simulink model "Solar_Seguidor_V2"  (R2021b)
settings: Solver=ode1  StartTime=0.0  StopTime=10  FixedStep=25e-6  RelTol=1e-3
PostLoadFcn:
  | %clc; clear all; close all;
  | %%%%%%%%%%%%%%%%%%%%%%%%%%%%%%%%%%%%%%%%%%%%%%%%
  | %%%%%%%%% Solar seguidor de rede %%%%%%%%%%
  | %%%%%%%%%%%%%%%%%%%%%%%%%%%%%%%%%%%%%%%%%%%%%%%%
  | %%%% Nominal Parameters %%%%
  | Pnom = 16e3;                                         % Potencia Nominal
  | Vnom_rms = 210;                                    % V linha rms
  | Vnom_peak = sqrt(2/3)*Vnom_rms;                     % V fase pico
  | FP_min = 1;                                       % Para suporte de reativo
  | Snom = Pnom/FP_min;                                 % Potencia aparente
  | Irms = Pnom/(sqrt(3)*Vnom_rms);                     % Ig rms
  | Inom_peak = Irms*sqrt(2);                           % Ig pico
  | Zbase = Vnom_peak/Inom_peak;                        % Impedancia Base
  | f = 60;                                             % Freq nominal
  | wnom = 2*pi*60;                                     % Freq Ang. nominal
  | m = 0.805;                                            % Indice mod nominal
  | Vdc = 2*(Vnom_peak/m);                              % Vcc
  | Vdc_2 = Vdc/2;                                      % Metade Vcc
  | Kconv = Zbase;                                      % Ganho conversor
  | %%%% Transformer %%%%
  | S_trafo = 250e3;                                      % transformer apparent power
  | Vrms_high = 400;                                   % transformer secondary voltage - Wye connection
  | Vrms_low = 210;                                   % transformer primary voltage - Delta connection
  | N = Vrms_high/Vrms_low;                             % transformation relationship
  | X_pu_trafo = 0.03;                                 % transformer p.u. reactance
  | Zb_trafo_high = ((Vrms_high)^2)/S_trafo;            % secondary base impedance
  | Zb_trafo = ((Vnom_rms)^2)/S_trafo;                  % primary base impedance
  | L_trafo = (X_pu_trafo*Zb_trafo)/wnom;               % primary inductance
  | %%%% LCL Filter Project %%%%
  | fsw = 105*60;%105*60;                                         % switching frequency
  | ripple = 0.05;                                       % current ripple
  | L1 = Vdc/(6*ripple*Inom_peak*fsw);                  % inductor L1
  |  RL1 = 0.005;                                        % L1 resistance
  |  Cbase = 1/(wnom*Kconv);                             % base capacitance
  |  Cf = 0.05*Cbase;                                    % filter capacitor
  | % Calculo do filtro
  | Sbase = 16e3;
  | %Sbase = 200e3*1.12;
  | V_LL = 210;
  | V_LG = 210/sqrt(3);
  | Vbase = V_LG*sqrt(2);
  | Ibase = (Sbase*sqrt(2))/(V_LG*3)*sqrt(3/2);
  | Zbase = (V_LL^2)/Sbase;
  | Rbase = Zbase;
  | Xbase = Zbase;
  | Lbase = Xbase/(2*pi*60);
  | Cbase = 1/(Xbase*2*pi*60);
  | w = 2*pi*60;
  | Q = 70;
  | Lf = 0.15*Lbase;
  | Cf = 0.05*Cbase;
  | fc = 1/(2*pi*sqrt(Lf*Cf));
  | R = (w*Lf)/Q;
  | Lf = L1;
  | R = RL1;
  | ka=0.2;                                             % attenuation factor
  | L2 = (sqrt(1/(ka^2))+1)/(Cf*((2*pi*fsw)^2));        % inductor L2
  | RL2 = 0.005;                                        % L2 resistance
  | w_res = sqrt((L1+L2+L_trafo)/(L1*L2*Cf));           % resonant angular frequency
  | f_res = w_res/(2*pi);                               % resonant frequency
  | ... (+31 lines)
InitFcn:
  | %clc; clear all; close all;
  | %%%%%%%%%%%%%%%%%%%%%%%%%%%%%%%%%%%%%%%%%%%%%%%%
  | %%%%%%%%% Solar seguidor de rede %%%%%%%%%%
  | %%%%%%%%%%%%%%%%%%%%%%%%%%%%%%%%%%%%%%%%%%%%%%%%
  | %%%% Nominal Parameters %%%%
  | Pnom = 16e3;                                         % Potencia Nominal
  | Vnom_rms = 210;                                    % V linha rms
  | Vnom_peak = sqrt(2/3)*Vnom_rms;                     % V fase pico
  | FP_min = 1;                                       % Para suporte de reativo
  | Snom = Pnom/FP_min;                                 % Potencia aparente
  | Irms = Pnom/(sqrt(3)*Vnom_rms);                     % Ig rms
  | Inom_peak = Irms*sqrt(2);                           % Ig pico
  | Zbase = Vnom_peak/Inom_peak;                        % Impedancia Base
  | f = 60;                                             % Freq nominal
  | wnom = 2*pi*60;                                     % Freq Ang. nominal
  | m = 0.805;                                            % Indice mod nominal
  | Vdc = 2*(Vnom_peak/m);                              % Vcc
  | Vdc_2 = Vdc/2;                                      % Metade Vcc
  | Kconv = Zbase;                                      % Ganho conversor
  | %%%% Transformer %%%%
  | S_trafo = 250e3;                                      % transformer apparent power
  | Vrms_high = 400;                                   % transformer secondary voltage - Wye connection
  | Vrms_low = 210;                                   % transformer primary voltage - Delta connection
  | N = Vrms_high/Vrms_low;                             % transformation relationship
  | X_pu_trafo = 0.03;                                 % transformer p.u. reactance
  | Zb_trafo_high = ((Vrms_high)^2)/S_trafo;            % secondary base impedance
  | Zb_trafo = ((Vnom_rms)^2)/S_trafo;                  % primary base impedance
  | L_trafo = (X_pu_trafo*Zb_trafo)/wnom;               % primary inductance
  | %%%% LCL Filter Project %%%%
  | fsw = 105*60;%105*60;                                         % switching frequency
  | ripple = 0.05;                                       % current ripple
  | L1 = Vdc/(6*ripple*Inom_peak*fsw);                  % inductor L1
  |  RL1 = 0.005;                                        % L1 resistance
  |  Cbase = 1/(wnom*Kconv);                             % base capacitance
  |  Cf = 0.05*Cbase;                                    % filter capacitor
  | % Calculo do filtro
  | Sbase = 16e3;
  | %Sbase = 200e3*1.12;
  | V_LL = 210;
  | V_LG = 210/sqrt(3);
  | Vbase = V_LG*sqrt(2);
  | Ibase = (Sbase*sqrt(2))/(V_LG*3)*sqrt(3/2);
  | Zbase = (V_LL^2)/Sbase;
  | Rbase = Zbase;
  | Xbase = Zbase;
  | Lbase = Xbase/(2*pi*60);
  | Cbase = 1/(Xbase*2*pi*60);
  | w = 2*pi*60;
  | Q = 70;
  | Lf = 0.15*Lbase;
  | Cf = 0.05*Cbase;
  | fc = 1/(2*pi*sqrt(Lf*Cf));
  | R = (w*Lf)/Q;
  | Lf = L1;
  | R = RL1;
  | ka=0.2;                                             % attenuation factor
  | L2 = (sqrt(1/(ka^2))+1)/(Cf*((2*pi*fsw)^2));        % inductor L2
  | RL2 = 0.005;                                        % L2 resistance
  | w_res = sqrt((L1+L2+L_trafo)/(L1*L2*Cf));           % resonant angular frequency
  | f_res = w_res/(2*pi);                               % resonant frequency
  | ... (+31 lines)
undefined symbols (not defined in the file): D1, Delta, DERS_models, DiscIntNeverNeededParam, eHS, I, Ia_PV, Ib_PV, Ic_PV, Left, parameter_set_id, ph, PV_system, type, V, Va_grid, Vb_grid, Vc_grid
libraries: powerlib_meascontrol x17, rtlab x14, spsThreePhaseSeriesRLCBranchLib x9, spsCurrentMeasurementLib x9, artemis x7, spsThreePhaseVIMeasurementLib x6, slpidlib x6, rteventslib x6, spsabctodq0Lib x4, spsThreePhaseTransformerTwoWindingsLib x3, simulink x3, spsPVArrayLib x3
(part 4 of 4)

== system Solar_Seguidor_V2/SM_mestre1/PV_system2/VSC_Control/Voltage DC Controller ==
  note: Voltage Controller
  Vdc_mes : Inport  PortDimensions=1
  Vdc_ref : Inport  Port=2  PortDimensions=1
  hab : Inport  Port=3
  Id_refm : Scope
  Math Function1 : Math  Operator=square  SaturateOnIntegerOverflow=on
  Math Function2 : Math  Commented=on  Operator=square  SaturateOnIntegerOverflow=on
  Math Function3 : Math  Operator=square  SaturateOnIntegerOverflow=on
  Mux : Mux  Inputs=2
  PI : slpidlib/PID Controller  Commented=on  Controller=PI  Form=Parallel  TimeDomain=Continuous-time  UseExternalTs=off  SampleTime=Ts  IntegratorMethod=Trapezoidal  FilterMethod=Forward Euler  ControllerParametersSource=internal  P=Kp_dc  I=ki_dc_pu  D=0  UseFilter=on  N=100  TunerSelectOption=Transfer Function Based (PID Tuner App)  InitialConditionSource=internal  InitialConditionForIntegrator=0  InitialConditionForFilter=0  DifferentiatorICPrevScaledInput=0  ExternalReset=rising  TrackingMode=off  Kt=1  LimitOutput=on  SatLimitsSource=internal  UpperSaturationLimit=1.4  LowerSaturationLimit=-2  LinearizeAsGain=off  AntiWindupMode=clamping  Kb=1  POutMin=[]  POutMax=[]  IOutMin=[]  IOutMax=[]  DOutMin=[]  DOutMax=[]  NOutMin=[]  NOutMax=[]  SumOutMin=[]  SumOutMax=[]  SaturationOutMin=[]  SaturationOutMax=[]  PParamMin=[]  PParamMax=[]  IParamMin=[]  IParamMax=[]  DParamMin=[]  DParamMax=[]  NParamMin=[]  NParamMax=[]  KbParamMin=[]  KbParamMax=[]  KtParamMin=[]  KtParamMax=[]  KbOutMin=[]  KbOutMax=[]  KtOutMin=[]  KtOutMax=[]  IntegratorOutMin=[]  IntegratorOutMax=[]  FilterOutMin=[]  FilterOutMax=[]  SumI1OutMin=[]  SumI1OutMax=[]  SumI2OutMin=[]  SumI2OutMax=[]  SumI3OutMin=[]  SumI3OutMax=[]  SumI4OutMin=[]  SumI4OutMax=[]  SumDOutMin=[]  SumDOutMax=[]  DifferentiatorOutMin=[]  DifferentiatorOutMax=[]  FilterDiffOutCoefMin=[]  FilterDiffOutCoefMax=[]  ReciprocalOutMin=[]  ReciprocalOutMax=[]  SumDenOutMin=[]  SumDenOutMax=[]  SumNumOutMin=[]  SumNumOutMax=[]  DivideOutMin=[]  DivideOutMax=[]  UdiffTsProdOutMin=[]  UdiffTsProdOutMax=[]  NTsProdOutMin=[]  NTsProdOutMax=[]  UintegralTsProdOutMin=[]  UintegralTsProdOutMax=[]  UngainTsProdOutMin=[]  UngainTsProdOutMax=[]  FilterDenConstantOutDataTypeStr=Inherit: Inherit via back propagation  FilterDenConstantOutMin=[]  FilterDenConstantOutMax=[]  PCopyOutDataTypeStr=Inherit: Inherit via back propagation  PCopyOutMin=[]  PCopyOutMax=[]  NCopyOutDataTypeStr=Inherit: Inherit via back propagation  NCopyOutMin=[]  NCopyOutMax=[]  IntegratorContinuousStateAttributes=''  IntegratorStateMustResolveToSignalObject=off  IntegratorRTWStateStorageClass=Auto  FilterContinuousStateAttributes=''  FilterStateMustResolveToSignalObject=off  FilterRTWStateStorageClass=Auto  ParallelPVariant=InternalParameters  IdealPVariant=Disabled  IVariant=InternalParameters  DVariant=Disabled  IntegratorVariant=Continuous  SatVariant=Enabled  AWVariant=ContClampingParallel  PCopyVariant=Disabled  TRVariant=Disabled  FdbkBlocksVariant=Forward  IdealPFdbkVariant=Disabled  SatFdbkVariant=Disabled  DerivativeFilterVariant=Disabled  NVariant=Disabled  NCopyVariant=Disabled_SignalSpec  FilterICVariant=Disabled  IntegratorICVariant=InternalICs  ExternalResetVariant=ExternalReset  TRSumVariant=Passthrough  SumFdbkVariant=Disabled  SumVariant=Sum_PI  TsampFilterVariant=InternalTs  TsampNgainVariant=Passthrough  TsampIntegralVariant=Passthrough  ExternalSaturationOutDataTypeStr=Inherit: Same as second input
  PI_Vdc2 : Subsystem
  Product : Product
  Rtot_pu1 : Gain  Gain=1/430  SaturateOnIntegerOverflow=on  OutDataTypeStr=Inherit: Same as input  ParamDataTypeStr=Inherit: Same as input
  Rtot_pu2 : Gain  Gain=1/430  SaturateOnIntegerOverflow=on  OutDataTypeStr=Inherit: Same as input  ParamDataTypeStr=Inherit: Same as input
  Rtot_pu3 : Gain  Gain=-1  SaturateOnIntegerOverflow=on  OutDataTypeStr=Inherit: Same as input  ParamDataTypeStr=Inherit: Same as input
  Saturation : Saturate  UpperLimit=1.2  LowerLimit=0
  Sum : Sum  Inputs=|-+
  Transfer Fcn2 : TransferFcn  Denominator=[2.53e-4 1]
  Voltage_DC : Scope
  Id_ref : Outport  SampleTime=Ts  InitialOutput=0  VectorParamsAs1DForOutWhenUnconnected=off
  wires:
  Saturation/1 -> Id_ref/1
  Vdc_mes/1 -> Transfer Fcn2/1
  Math Function3/1 -> Sum/2
  Math Function1/1 -> Sum/1
  Rtot_pu2/1 -> Math Function3/1, Mux/2
  Rtot_pu1/1 -> Math Function1/1, Mux/1
  Mux/1 -> Voltage_DC/1
  hab/1 -> Product/2, PI_Vdc2/2(hab)
  Sum/1 -> Rtot_pu3/1
  Vdc_ref/1 -> Rtot_pu2/1
  Rtot_pu3/1 -> PI_Vdc2/1(e_Vdc)
  Transfer Fcn2/1 -> Rtot_pu1/1
  PI_Vdc2/1(u) -> Product/1
  Product/1 -> Id_refm/1, Saturation/1

== system Solar_Seguidor_V2/SM_mestre1/PV_system/VSC_Control/Maximum Power Point/MPPT Parameters ==
  Lower limit for Vdc_ref (Dmax) : Constant  Value=375
  Mux9 : Mux
  Upper limit for Vdc_ref (Dmax : Constant  Value=430
  Vdc_ref (DeltaD) : Constant  Value=3e-4*0.5
  Vdc_ref output (Dinit) : Constant  Value=425
  Param : Outport  VectorParamsAs1DForOutWhenUnconnected=off
  wires:
  Upper limit for Vdc_ref (Dmax/1 -> Mux9/2
  Lower limit for Vdc_ref (Dmax)/1 -> Mux9/3
  Vdc_ref output (Dinit)/1 -> Mux9/1
  Mux9/1 -> Param/1
  Vdc_ref (DeltaD)/1 -> Mux9/4

== system Solar_Seguidor_V2/SM_mestre1/PV_system/VSC_Control/PLL & dq/Subsystem ==
  wt : Inport
  Vabc : Inport  Port=2
  Iabc : Inport  Port=3
  Demux : Demux  Outputs=3
  Demux1 : Demux  Outputs=3
  Gain : Gain  Gain=3/2
  Gain1 : Gain  Gain=1/1e3
  Product : Product
  Product1 : Product
  Sum : Sum
  Transfer Fcn : TransferFcn  Denominator=[3/4 1]
  abc to dq1 : powerlib_meascontrol/Transformations/abc to dq0  Alignment=90 degrees behind phase A axis
  abc to dq2 : powerlib_meascontrol/Transformations/abc to dq0  Alignment=90 degrees behind phase A axis
  P_PV : Outport
  wires:
  [Id] -> Product/2
  Product/1 -> Sum/1
  Gain1/1 -> Transfer Fcn/1
  [Vd] -> Product/1
  Gain/1 -> Gain1/1
  [Iq] -> Product1/2
  Sum/1 -> Gain/1
  Product1/1 -> Sum/2
  Transfer Fcn/1 -> P_PV/1
  [Vq] -> Product1/1
  Vabc/1 -> abc to dq1/1
  wt/1 -> abc to dq2/2, abc to dq1/2
  Iabc/1 -> abc to dq2/1
  abc to dq1/1 -> Demux/1
  Demux/1 -> [Vd]
  Demux/2 -> [Vq]
  Demux1/2 -> [Iq]
  Demux1/1 -> [Id]
  abc to dq2/1 -> Demux1/1

== system Solar_Seguidor_V2/SM_mestre1/PV_system1/VSC_Control/Maximum Power Point/MPPT Parameters ==
  Lower limit for Vdc_ref (Dmax) : Constant  Value=375
  Mux9 : Mux
  Upper limit for Vdc_ref (Dmax : Constant  Value=430
  Vdc_ref (DeltaD) : Constant  Value=3e-4*0.5
  Vdc_ref output (Dinit) : Constant  Value=425
  Param : Outport  VectorParamsAs1DForOutWhenUnconnected=off
  wires:
  Vdc_ref (DeltaD)/1 -> Mux9/4
  Mux9/1 -> Param/1
  Vdc_ref output (Dinit)/1 -> Mux9/1
  Lower limit for Vdc_ref (Dmax)/1 -> Mux9/3
  Upper limit for Vdc_ref (Dmax/1 -> Mux9/2

== system Solar_Seguidor_V2/SM_mestre1/PV_system1/VSC_Control/PLL & dq/Subsystem ==
  wt : Inport
  Vabc : Inport  Port=2
  Iabc : Inport  Port=3
  Demux : Demux  Outputs=3
  Demux1 : Demux  Outputs=3
  Gain : Gain  Gain=3/2
  Gain1 : Gain  Gain=1/1e3
  Product : Product
  Product1 : Product
  Sum : Sum
  Transfer Fcn : TransferFcn  Denominator=[3/4 1]
  abc to dq1 : powerlib_meascontrol/Transformations/abc to dq0  Alignment=90 degrees behind phase A axis
  abc to dq2 : powerlib_meascontrol/Transformations/abc to dq0  Alignment=90 degrees behind phase A axis
  P_PV : Outport
  wires:
  abc to dq2/1 -> Demux1/1
  Demux1/1 -> [Id]
  Demux1/2 -> [Iq]
  Demux/2 -> [Vq]
  Demux/1 -> [Vd]
  abc to dq1/1 -> Demux/1
  Iabc/1 -> abc to dq2/1
  wt/1 -> abc to dq1/2, abc to dq2/2
  Vabc/1 -> abc to dq1/1
  [Vq] -> Product1/1
  Transfer Fcn/1 -> P_PV/1
  Product1/1 -> Sum/2
  Sum/1 -> Gain/1
  [Iq] -> Product1/2
  Gain/1 -> Gain1/1
  [Vd] -> Product/1
  Gain1/1 -> Transfer Fcn/1
  Product/1 -> Sum/1
  [Id] -> Product/2

== system Solar_Seguidor_V2/SM_mestre1/PV_system2/VSC_Control/Current Controller/PI_Idq1 ==
  e_Idq : Inport
  hab : Inport  Port=2
  Discrete-Time Integrator : DiscreteIntegrator  SampleTime=-1  ICPrevOutput=DiscIntNeverNeededParam  ICPrevScaledInput=DiscIntNeverNeededParam
  Gain1 : Gain  Gain=kp_current_pu
  Gain2 : Gain  Gain=ki_current_pu
  Product : Product
  Sum1 : Sum
  u : Outport
  wires:
  hab/1 -> Product/2
  e_Idq/1 -> Product/1
  Discrete-Time Integrator/1 -> Sum1/2
  Sum1/1 -> u/1
  Gain1/1 -> Sum1/1
  Product/1 -> Gain2/1, Gain1/1
  Gain2/1 -> Discrete-Time Integrator/1

== system Solar_Seguidor_V2/SM_mestre1/PV_system2/VSC_Control/Maximum Power Point/MPPT Parameters ==
  Lower limit for Vdc_ref (Dmax) : Constant  Value=375
  Mux9 : Mux
  Upper limit for Vdc_ref (Dmax : Constant  Value=430
  Vdc_ref (DeltaD) : Constant  Value=3e-4*0.5
  Vdc_ref output (Dinit) : Constant  Value=425
  Param : Outport  VectorParamsAs1DForOutWhenUnconnected=off
  wires:
  Vdc_ref (DeltaD)/1 -> Mux9/4
  Mux9/1 -> Param/1
  Vdc_ref output (Dinit)/1 -> Mux9/1
  Lower limit for Vdc_ref (Dmax)/1 -> Mux9/3
  Upper limit for Vdc_ref (Dmax/1 -> Mux9/2

== system Solar_Seguidor_V2/SM_mestre1/PV_system2/VSC_Control/PLL & dq/Subsystem ==
  wt : Inport
  Vabc : Inport  Port=2
  Iabc : Inport  Port=3
  Demux : Demux  Outputs=3
  Demux1 : Demux  Outputs=3
  Gain : Gain  Gain=3/2
  Gain1 : Gain  Gain=1/1e3
  Product : Product
  Product1 : Product
  Sum : Sum
  Transfer Fcn : TransferFcn  Denominator=[3/4 1]
  abc to dq1 : spsabctodq0Lib/abc to dq0  Alignment=90 degrees behind phase A axis
  abc to dq2 : spsabctodq0Lib/abc to dq0  Alignment=90 degrees behind phase A axis
  P_PV : Outport
  wires:
  abc to dq2/1 -> Demux1/1
  Demux1/1 -> [Id]
  Demux1/2 -> [Iq]
  Demux/2 -> [Vq]
  Demux/1 -> [Vd]
  abc to dq1/1 -> Demux/1
  Iabc/1 -> abc to dq2/1
  wt/1 -> abc to dq1/2, abc to dq2/2
  Vabc/1 -> abc to dq1/1
  [Vq] -> Product1/1
  Transfer Fcn/1 -> P_PV/1
  Product1/1 -> Sum/2
  Sum/1 -> Gain/1
  [Iq] -> Product1/2
  Gain/1 -> Gain1/1
  [Vd] -> Product/1
  Gain1/1 -> Transfer Fcn/1
  Product/1 -> Sum/1
  [Id] -> Product/2

== system Solar_Seguidor_V2/SM_mestre1/PV_system2/VSC_Control/Voltage DC Controller/PI_Vdc2 ==
  e_Vdc : Inport
  hab : Inport  Port=2
  Discrete-Time Integrator : DiscreteIntegrator  SampleTime=-1  ICPrevOutput=DiscIntNeverNeededParam  ICPrevScaledInput=DiscIntNeverNeededParam
  Gain1 : Gain  Gain=Kp_dc
  Gain2 : Gain  Gain=ki_dc_pu
  Product : Product
  Sum1 : Sum
  u : Outport
  wires:
  Gain2/1 -> Discrete-Time Integrator/1
  Product/1 -> Gain1/1, Gain2/1
  Gain1/1 -> Sum1/1
  Sum1/1 -> u/1
  Discrete-Time Integrator/1 -> Sum1/2
  e_Vdc/1 -> Product/1
  hab/1 -> Product/2

== matlab function Solar_Seguidor_V2/SM_mestre1/PV_system/VSC_Control/Maximum Power Point/MPPT Controller using Perturbe & Observe technique 2 ==
  settings: updateMethod=DISCRETE  sampleTime=Ts*2
  data: Param input; Enabled input; V input; I input; D output
function D  = PandO(Param, Enabled, V, I)

% MPPT controller based on the Perturb & Observe algorithm.

% D output = Reference for DC link voltage (Vdc_ref) 
%
% Enabled input = 1 to enable the MPPT controller
% V input = PV array terminal voltage (V)
% I input = PV array current (A)
%
% Param input:
Dinit = Param(1);  %Initial value for Vdc_ref
Dmax = Param(2);   %Maximum value for Vdc_ref
Dmin = Param(3);   %Minimum value for Vdc_ref
deltaD = Param(4); %Increment value used to increase/decrease Vdc_ref
%  

persistent Vold Pold Dold;

dataType = 'double';

if isempty(Vold)
    Vold=0;
    Pold=0;
    Dold=Dinit;
end
P= V*I;
dV= V - Vold;
dP= P - Pold;

if dP ~= 0 & Enabled ~=0
    if dP < 0
        if dV < 0
            D = Dold + deltaD;
        else
            D = Dold - deltaD;
        end
    else
        if dV < 0
            D = Dold - deltaD;
        else
            D = Dold + deltaD;
        end    
    end
else D=Dold;
end

if D >= Dmax | D<= Dmin
    D=Dold;
end

Dold=D;
Vold=V;
Pold=P;

== matlab function Solar_Seguidor_V2/SM_mestre1/PV_system1/VSC_Control/Maximum Power Point/MPPT Controller using Perturbe & Observe technique 2 ==
  settings: updateMethod=DISCRETE  sampleTime=Ts*2
  data: Param input; Enabled input; V input; I input; D output
function D  = PandO(Param, Enabled, V, I)

% MPPT controller based on the Perturb & Observe algorithm.

% D output = Reference for DC link voltage (Vdc_ref) 
%
% Enabled input = 1 to enable the MPPT controller
% V input = PV array terminal voltage (V)
% I input = PV array current (A)
%
% Param input:
Dinit = Param(1);  %Initial value for Vdc_ref
Dmax = Param(2);   %Maximum value for Vdc_ref
Dmin = Param(3);   %Minimum value for Vdc_ref
deltaD = Param(4); %Increment value used to increase/decrease Vdc_ref
%  

persistent Vold Pold Dold;

dataType = 'double';

if isempty(Vold)
    Vold=0;
    Pold=0;
    Dold=Dinit;
end
P= V*I;
dV= V - Vold;
dP= P - Pold;

if dP ~= 0 & Enabled ~=0
    if dP < 0
        if dV < 0
            D = Dold + deltaD;
        else
            D = Dold - deltaD;
        end
    else
        if dV < 0
            D = Dold - deltaD;
        else
            D = Dold + deltaD;
        end    
    end
else D=Dold;
end

if D >= Dmax | D<= Dmin
    D=Dold;
end

Dold=D;
Vold=V;
Pold=P;

== matlab function Solar_Seguidor_V2/SM_mestre1/PV_system2/VSC_Control/Maximum Power Point/MPPT Controller using Perturbe & Observe technique 2 ==
  settings: updateMethod=DISCRETE  sampleTime=Ts*2
  data: Param input; Enabled input; V input; I input; D output
function D  = PandO(Param, Enabled, V, I)

% MPPT controller based on the Perturb & Observe algorithm.

% D output = Reference for DC link voltage (Vdc_ref) 
%
% Enabled input = 1 to enable the MPPT controller
% V input = PV array terminal voltage (V)
% I input = PV array current (A)
%
% Param input:
Dinit = Param(1);  %Initial value for Vdc_ref
Dmax = Param(2);   %Maximum value for Vdc_ref
Dmin = Param(3);   %Minimum value for Vdc_ref
deltaD = Param(4); %Increment value used to increase/decrease Vdc_ref
%  

persistent Vold Pold Dold;

dataType = 'double';

if isempty(Vold)
    Vold=0;
    Pold=0;
    Dold=Dinit;
end
P= V*I;
dV= V - Vold;
dP= P - Pold;

if dP ~= 0 & Enabled ~=0
    if dP < 0
        if dV < 0
            D = Dold + deltaD;
        else
            D = Dold - deltaD;
        end
    else
        if dV < 0
            D = Dold - deltaD;
        else
            D = Dold + deltaD;
        end    
    end
else D=Dold;
end

if D >= Dmax | D<= Dmin
    D=Dold;
end

Dold=D;
Vold=V;
Pold=P;
